simulink library "actuator_processing"  (R2016b)
settings: Solver=VariableStepAuto  StartTime=0.0  StopTime=10.0  RelTol=1e-3
settings Model: Creator=taylorreynolds  LastModifiedBy=Taylor

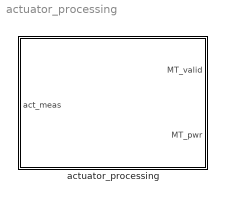
== system actuator_processing ==
  actuator_processing : Subsystem

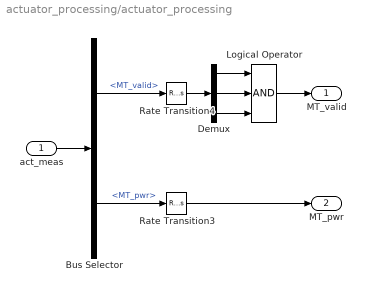
== system actuator_processing/actuator_processing ==
  act_meas : Inport
  Bus Selector : BusSelector  OutputSignals=MT_valid,MT_pwr
  Demux : Demux  Outputs=[1 1 1]
  Logical Operator : Logic  Inputs=3  AllPortsSameDT=off  OutDataTypeStr=boolean
  Rate Transition3 : RateTransition  OutPortSampleTime=fsw_params.sample_time_s
  Rate Transition4 : RateTransition  OutPortSampleTime=fsw_params.sample_time_s
  MT_valid : Outport
  MT_pwr : Outport  Port=2
  wires:
  Bus Selector/2 -> Rate Transition3/1  "<MT_pwr>"
  Bus Selector/1 -> Rate Transition4/1  "<MT_valid>"
  act_meas/1 -> Bus Selector/1
  Rate Transition4/1 -> Demux/1
  Rate Transition3/1 -> MT_pwr/1
  Demux/2 -> Logical Operator/2
  Demux/1 -> Logical Operator/1
  Demux/3 -> Logical Operator/3
  Logical Operator/1 -> MT_valid/1
